simulink model "sampleModel1949"  (R2023a)
settings: Solver=VariableStepAuto  StartTime=0.0  StopTime=10.0  RelTol=1e-3
libraries: hdlsllib x6
settings Model: Creator=user1  LastModifiedBy=user1

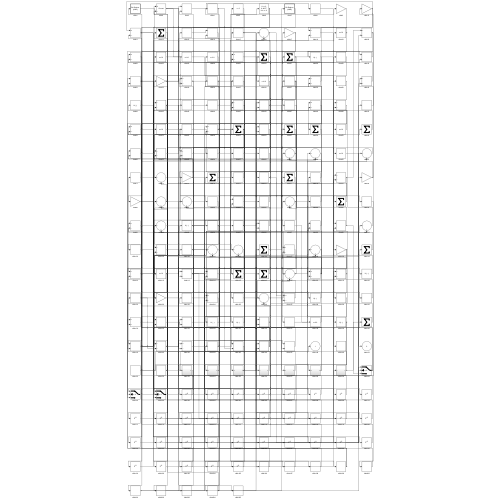
[thumbnail: Simulink's stored preview of the top-level diagram]
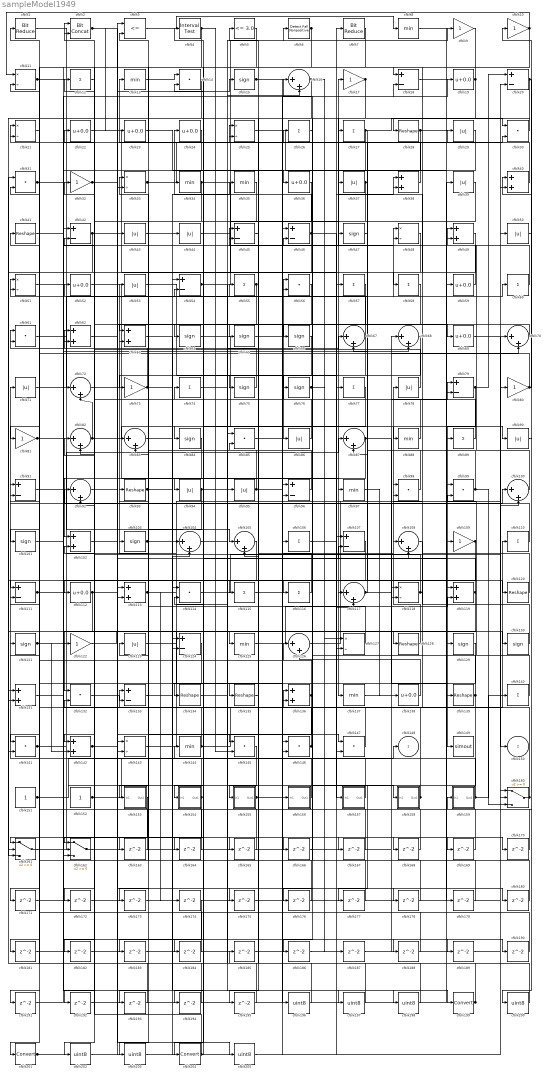
== system sampleModel1949 ==
  cfblk1 : hdlsllib/Logic and Bit Operations/Bit Reduce  mode=AND
  cfblk{9..10,17,32,73,80..81,109,122} (9 alike) : Gain
  cfblk{16,67..68,70,72,82..83,87,92,100,104..105,108,117,126} (15 alike) : Sum  Inputs=|++
  cfblk{15,47,64..66,75..76,84,101,103,121,129..130} (13 alike) : Signum
  cfblk{38,40,49,62..63,102,113,119,131,136,142} (11 alike) : Sum
  cfblk{12,26..27,55,57..58,60,74,77,89,106,110,115..116,140} (15 alike) : Sum  Inputs=+
  cfblk{18,20,42,45..46,54,79,91,96,107,111,124,133} (13 alike) : Sum  Inputs=+-
  cfblk{11,21,25,33,48,51,118,127,143} (9 alike) : Product  Inputs=*/  RndMeth=Zero  SaturateOnIntegerOverflow=on
  cfblk{19,22..24,36,52,59,69,112,138} (10 alike) : Bias  Bias=0.0  SaturateOnIntegerOverflow=off
  cfblk{14,30..31,56,61,85,98..99,114,132,141,145..147} (14 alike) : DotProduct  OutDataTypeStr=Inherit: Inherit via internal rule
  cfblk{28,41,93,120,128,134..135,139} (8 alike) : Reshape
  cfblk{29,37,39,43..44,50,53,71,78,86,90,94..95,123} (14 alike) : Abs  SaturateOnIntegerOverflow=off
  cfblk{8,13,34..35,88,97,125,137,144} (9 alike) : MinMax
  cfblk149 : ToWorkspace  VariableName=simout  SaveFormat=Timeseries  SampleTime=-1
  cfblk151 : Constant  SampleTime=-1
  cfblk152 : Constant  SampleTime=-1
  cfblk153 : Subsystem
      settings: LibrarySourceBlock=|
      | hdlsllib/Ports &
      | Subsystems/Subsystem
  cfblk154 : Subsystem
      settings: LibrarySourceBlock=|
      | hdlsllib/Ports &
      | Subsystems/Subsystem
  cfblk155 : Subsystem
      settings: LibrarySourceBlock=|
      | hdlsllib/Ports &
      | Subsystems/Subsystem
  cfblk156 : Subsystem
      settings: LibrarySourceBlock=|
      | hdlsllib/Ports &
      | Subsystems/Subsystem
  cfblk157 : Subsystem
      settings: LibrarySourceBlock=|
      | hdlsllib/Ports &
      | Subsystems/Subsystem
  cfblk158 : Subsystem
      settings: LibrarySourceBlock=|
      | hdlsllib/Ports &
      | Subsystems/Subsystem
  cfblk159 : Subsystem
      settings: LibrarySourceBlock=|
      | hdlsllib/Ports &
      | Subsystems/Subsystem
  cfblk160 : Switch  SaturateOnIntegerOverflow=off  InputSameDT=off
  cfblk161 : Switch  SaturateOnIntegerOverflow=off  InputSameDT=off
  cfblk162 : Switch  SaturateOnIntegerOverflow=off  InputSameDT=off
  cfblk{163..195} (33 alike) : Delay  SampleTime=1
  cfblk{196..198,200,202..203,205} (7 alike) : DataTypeConversion  OutDataTypeStr=uint8  SaturateOnIntegerOverflow=off  RndMeth=Floor
  cfblk199 : DataTypeConversion  SaturateOnIntegerOverflow=off  RndMeth=Floor
  cfblk2 : hdlsllib/Logic and Bit Operations/Bit Concat  numInputs=2
  cfblk201 : DataTypeConversion  SaturateOnIntegerOverflow=off  RndMeth=Floor
  cfblk204 : DataTypeConversion  SaturateOnIntegerOverflow=off  RndMeth=Floor
  cfblk3 : RelationalOperator  Operator=<=  OutDataTypeStr=boolean  InputSameDT=off
  cfblk4 : hdlsllib/Logic and Bit Operations/Interval Test  IntervalClosedRight=on  uplimit=0.5  IntervalClosedLeft=on  lowlimit=-0.5  OutDataTypeStr=boolean
  cfblk5 : hdlsllib/Logic and Bit Operations/Compare To Constant  relop=<=  const=3.0  OutDataTypeStr=boolean
  cfblk6 : hdlsllib/Logic and Bit Operations/Detect Fall Nonpositive  vinit=0  OutDataTypeStr=boolean
  cfblk7 : hdlsllib/Logic and Bit Operations/Bit Reduce  mode=AND
  cfblk148 : Outport  VectorParamsAs1DForOutWhenUnconnected=off
  cfblk150 : Outport  Port=2  VectorParamsAs1DForOutWhenUnconnected=off
  wires:
  cfblk82/1 -> cfblk84/1, cfblk72/2
  cfblk154/1(Out1) -> cfblk161/1, cfblk93/1
  cfblk97/1 -> cfblk138/1
  cfblk157/1(Out1) -> cfblk71/1
  cfblk17/1 -> cfblk137/1, cfblk76/1
  cfblk46/1 -> cfblk24/1, cfblk130/1, cfblk111/1
  cfblk1/1 -> cfblk105/1
  cfblk141/1 -> cfblk87/1, cfblk18/2, cfblk30/2, cfblk136/1
  cfblk108/1 -> cfblk133/1
  cfblk43/1 -> cfblk44/1
  cfblk128/1 -> cfblk78/1
  cfblk84/1 -> cfblk102/1
  cfblk2/1 -> cfblk23/1, cfblk69/1, cfblk205/1
  cfblk88/1 -> cfblk56/1
  cfblk37/1 -> cfblk125/1, cfblk64/1, cfblk67/2
  cfblk38/1 -> cfblk13/1
  cfblk132/1 -> cfblk133/2
  cfblk72/1 -> cfblk97/1
  cfblk160/1 -> cfblk123/1, cfblk91/2
  cfblk49/1 -> cfblk94/1
  cfblk111/1 -> cfblk7/1, cfblk54/1
  cfblk52/1 -> cfblk90/1
  cfblk121/1 -> cfblk53/1, cfblk142/2
  cfblk145/1 -> cfblk155/1(In1)
  cfblk161/1 -> cfblk77/1
  cfblk98/1 -> cfblk52/1
  cfblk81/1 -> cfblk42/1, cfblk127/2
  cfblk124/1 -> cfblk201/1
  cfblk109/1 -> cfblk149/1, cfblk202/1
  cfblk54/1 -> cfblk6/1, cfblk89/1
  cfblk137/1 -> cfblk79/1
  cfblk122/1 -> cfblk135/1
  cfblk67/1 -> cfblk86/1, cfblk41/1
  cfblk22/1 -> cfblk156/1(In1)
  cfblk135/1 -> cfblk5/1
  cfblk126/1 -> cfblk80/1
  cfblk79/1 -> cfblk129/1, cfblk20/1
  cfblk10/1 -> cfblk11/1, cfblk58/1, cfblk194/1
  cfblk3/1 -> cfblk8/1
  cfblk64/1 -> cfblk88/1
  cfblk74/1 -> cfblk199/1
  cfblk153/1(Out1) -> cfblk162/1
  cfblk144/1 -> cfblk110/1, cfblk21/2
  cfblk47/1 -> cfblk117/1
  cfblk8/1 -> cfblk109/1
  cfblk16/1 -> cfblk81/1, cfblk127/1
  cfblk20/1 -> cfblk159/1(In1), cfblk145/1
  cfblk51/1 -> cfblk48/1
  cfblk125/1 -> cfblk119/2
  cfblk134/1 -> cfblk9/1
  cfblk114/1 -> cfblk50/1
  cfblk127/1 -> cfblk33/1
  cfblk6/1 -> cfblk73/1, cfblk191/1
  cfblk143/1 -> cfblk46/1
  cfblk63/1 -> cfblk104/1
  cfblk89/1 -> cfblk21/1
  cfblk33/1 -> cfblk29/1, cfblk83/2
  cfblk116/1 -> cfblk55/1
  cfblk129/1 -> cfblk134/1
  cfblk162/1 -> cfblk68/1
  cfblk110/1 -> cfblk91/1
  cfblk31/1 -> cfblk184/1, cfblk197/1
  cfblk107/1 -> cfblk154/1(In1)
  cfblk119/1 -> cfblk132/1, cfblk107/2
  cfblk71/1 -> cfblk48/2
  cfblk104/1 -> cfblk67/1
  cfblk23/1 -> cfblk36/1
  cfblk147/1 -> cfblk34/1
  cfblk105/1 -> cfblk131/2
  cfblk152/1 -> cfblk148/1, cfblk132/2
  cfblk19/1 -> cfblk18/1, cfblk181/1
  cfblk25/1 -> cfblk99/1
  cfblk96/1 -> cfblk61/1
  cfblk76/1 -> cfblk26/1, cfblk187/1
  cfblk75/1 -> cfblk22/1
  cfblk151/1 -> cfblk106/1, cfblk158/1(In1)
  cfblk60/1 -> cfblk17/1
  cfblk5/1 -> cfblk101/1
  cfblk94/1 -> cfblk153/1(In1), cfblk16/2
  cfblk53/1 -> cfblk107/1
  cfblk24/1 -> cfblk162/2
  cfblk155/1(Out1) -> cfblk108/1, cfblk98/1
  cfblk45/1 -> cfblk65/1
  cfblk61/1 -> cfblk60/1
  cfblk146/1 -> cfblk103/1, cfblk92/2
  cfblk156/1(Out1) -> cfblk62/1
  cfblk100/1 -> cfblk49/1
  cfblk27/1 -> cfblk56/2, cfblk30/1, cfblk87/2
  cfblk12/1 -> cfblk122/1
  cfblk80/1 -> cfblk40/1, cfblk51/1
  cfblk39/1 -> cfblk66/1
  cfblk55/1 -> cfblk172/1, cfblk173/1
  cfblk21/1 -> cfblk141/1
  cfblk69/1 -> cfblk150/1
  cfblk87/1 -> cfblk113/2, cfblk139/1
  cfblk118/1 -> cfblk62/2, cfblk98/2, cfblk54/2
  cfblk7/1 -> cfblk82/2
  cfblk93/1 -> cfblk118/2, cfblk35/1, cfblk168/1
  cfblk136/1 -> cfblk51/2, cfblk183/1
  cfblk106/1 -> cfblk38/1
  cfblk103/1 -> cfblk128/1, cfblk136/2
  cfblk78/1 -> cfblk2/1
  cfblk40/1 -> cfblk3/2
  cfblk139/1 -> cfblk92/1, cfblk176/1, cfblk177/1
  cfblk131/1 -> cfblk100/1
  cfblk44/1 -> cfblk47/1
  cfblk62/1 -> cfblk43/1
  cfblk30/1 -> cfblk28/1
  cfblk4/1 -> cfblk33/2, cfblk145/2
  cfblk138/1 -> cfblk126/2
  cfblk158/1(Out1) -> cfblk121/1, cfblk4/1
  cfblk113/1 -> cfblk39/1, cfblk147/2, cfblk174/1, cfblk175/1
  cfblk130/1 -> cfblk38/2
  cfblk42/1 -> cfblk143/2, cfblk141/2
  cfblk142/1 -> cfblk147/1, cfblk108/2
  cfblk50/1 -> cfblk10/1
  cfblk120/1 -> cfblk37/1
  cfblk73/1 -> cfblk31/2, cfblk190/1
  cfblk57/1 -> cfblk204/1
  cfblk34/1 -> cfblk157/1(In1), cfblk112/1
  cfblk11/1 -> cfblk68/2, cfblk120/1
  cfblk159/1(Out1) -> cfblk144/1, cfblk140/1
  cfblk123/1 -> cfblk95/1
  cfblk99/1 -> cfblk45/1, cfblk160/3
  cfblk86/1 -> cfblk32/1
  cfblk112/1 -> cfblk116/1, cfblk161/3
  cfblk66/1 -> cfblk115/1
  cfblk15/1 -> cfblk96/2, cfblk188/1
  cfblk9/1 -> cfblk162/3
  cfblk14/1 -> cfblk161/2
  cfblk28/1 -> cfblk59/1, cfblk182/1
  cfblk59/1 -> cfblk25/1
  cfblk70/1 -> cfblk63/1
  cfblk13/1 -> cfblk14/1
  cfblk117/1 -> cfblk70/2, cfblk27/1
  cfblk95/1 -> cfblk14/2, cfblk19/1
  cfblk32/1 -> cfblk15/1, cfblk25/2
  cfblk140/1 -> cfblk99/2
  cfblk56/1 -> cfblk142/1
  cfblk36/1 -> cfblk75/1
  cfblk68/1 -> cfblk163/1
  cfblk163/1 -> cfblk1/1
  cfblk77/1 -> cfblk164/1
  cfblk164/1 -> cfblk143/1
  cfblk102/1 -> cfblk165/1
  cfblk165/1 -> cfblk42/2
  cfblk83/1 -> cfblk166/1
  cfblk166/1 -> cfblk126/1
  cfblk101/1 -> cfblk167/1
  cfblk167/1 -> cfblk114/1
  cfblk168/1 -> cfblk46/2
  cfblk91/1 -> cfblk169/1
  cfblk169/1 -> cfblk96/1
  cfblk115/1 -> cfblk170/1
  cfblk170/1 -> cfblk113/1
  cfblk48/1 -> cfblk171/1
  cfblk171/1 -> cfblk79/2
  cfblk172/1 -> cfblk117/2
  cfblk173/1 -> cfblk40/2
  cfblk175/1 -> cfblk105/2
  cfblk176/1 -> cfblk61/2
  cfblk177/1 -> cfblk63/2
  cfblk92/1 -> cfblk178/1
  cfblk178/1 -> cfblk16/1
  cfblk18/1 -> cfblk179/1
  cfblk179/1 -> cfblk82/1
  cfblk65/1 -> cfblk180/1
  cfblk180/1 -> cfblk45/2
  cfblk181/1 -> cfblk160/2
  cfblk182/1 -> cfblk100/2
  cfblk183/1 -> cfblk104/2
  cfblk184/1 -> cfblk2/2
  cfblk185/1 -> cfblk20/2
  cfblk26/1 -> cfblk186/1
  cfblk186/1 -> cfblk118/1
  cfblk187/1 -> cfblk49/2
  cfblk188/1 -> cfblk11/2
  cfblk41/1 -> cfblk189/1
  cfblk189/1 -> cfblk70/1
  cfblk190/1 -> cfblk146/1
  cfblk191/1 -> cfblk72/1
  cfblk35/1 -> cfblk192/1
  cfblk192/1 -> cfblk119/1
  cfblk58/1 -> cfblk193/1
  cfblk193/1 -> cfblk3/1
  cfblk194/1 -> cfblk111/2
  cfblk29/1 -> cfblk195/1
  cfblk195/1 -> cfblk131/1
  cfblk85/1 -> cfblk196/1
  cfblk196/1 -> cfblk12/1
  cfblk197/1 -> cfblk85/1
  cfblk133/1 -> cfblk198/1
  cfblk198/1 -> cfblk85/2
  cfblk199/1 -> cfblk185/1, cfblk31/1
  cfblk90/1 -> cfblk200/1
  cfblk200/1 -> cfblk74/1
  cfblk201/1 -> cfblk146/2, cfblk83/1
  cfblk202/1 -> cfblk124/1
  cfblk174/1 -> cfblk203/1
  cfblk203/1 -> cfblk124/2
  cfblk204/1 -> cfblk160/1, cfblk114/2, cfblk102/2
  cfblk205/1 -> cfblk57/1

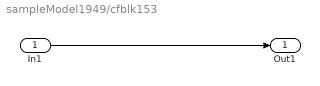
== system sampleModel1949/cfblk153 ==
  In1 : Inport
  Out1 : Outport
  wires:
  In1/1 -> Out1/1

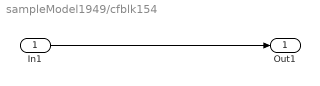
== system sampleModel1949/cfblk154 ==
  In1 : Inport
  Out1 : Outport
  wires:
  In1/1 -> Out1/1

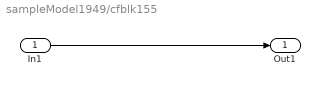
== system sampleModel1949/cfblk155 ==
  In1 : Inport
  Out1 : Outport
  wires:
  In1/1 -> Out1/1

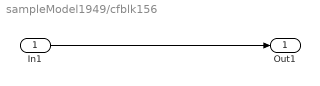
== system sampleModel1949/cfblk156 ==
  In1 : Inport
  Out1 : Outport
  wires:
  In1/1 -> Out1/1

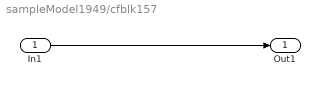
== system sampleModel1949/cfblk157 ==
  In1 : Inport
  Out1 : Outport
  wires:
  In1/1 -> Out1/1

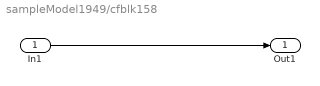
== system sampleModel1949/cfblk158 ==
  In1 : Inport
  Out1 : Outport
  wires:
  In1/1 -> Out1/1

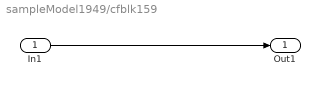
== system sampleModel1949/cfblk159 ==
  In1 : Inport
  Out1 : Outport
  wires:
  In1/1 -> Out1/1
